simulink model "transfer_function"  (R2023a)
settings: Solver=VariableStepAuto  StartTime=0.0  StopTime=t_simulation  RelTol=1e-3
values from neighbouring files (symbols this model uses):
  A_alpha = -.1    (= -0.1)    [main.m]
  A_beta = 10    [main.m]
  A_wind = -1    [main.m]
  bool_alpha = 0    [main.m]
  bool_beta = 0    [main.m]
  bool_wind = 0    [main.m]
  G_D_sim = table_tf(table_tf.wind_speed==v_wind,:).G_D    [main.m]
  G_D_sim_denominator_1 = table_tf(table_tf.wind_speed==v_wind,:).G_D_denominator{:}(1,1)    [main.m]
  G_D_sim_denominator_2 = table_tf(table_tf.wind_speed==v_wind,:).G_D_denominator{:}(2,1)    [main.m]
  G_D_sim_numerator_1 = table_tf(table_tf.wind_speed==v_wind,:).G_D_numerator{:}(1,1)    [main.m]
  G_D_sim_numerator_2 = table_tf(table_tf.wind_speed==v_wind,:).G_D_numerator{:}(2,1)    [main.m]
  G_S_sim = table_tf(table_tf.wind_speed==v_wind,:).G_S    [main.m]
  G_S_sim_denominator_11 = table_tf(table_tf.wind_speed==v_wind,:).G_S_denominator{:}(1,1)    [main.m]
  G_S_sim_denominator_12 = table_tf(table_tf.wind_speed==v_wind,:).G_S_denominator{:}(1,2)    [main.m]
  G_S_sim_denominator_21 = table_tf(table_tf.wind_speed==v_wind,:).G_S_denominator{:}(2,1)    [main.m]
  G_S_sim_denominator_22 = table_tf(table_tf.wind_speed==v_wind,:).G_S_denominator{:}(2,2)    [main.m]
  G_S_sim_numerator_11 = table_tf(table_tf.wind_speed==v_wind,:).G_S_numerator{:}(1,1)    [main.m]
  G_S_sim_numerator_12 = table_tf(table_tf.wind_speed==v_wind,:).G_S_numerator{:}(1,2)    [main.m]
  G_S_sim_numerator_21 = table_tf(table_tf.wind_speed==v_wind,:).G_S_numerator{:}(2,1)    [main.m]
  G_S_sim_numerator_22 = table_tf(table_tf.wind_speed==v_wind,:).G_S_numerator{:}(2,2)    [main.m]
  PID_11 = PID_Ziegler_Nichols(-G_11,t_linspace)    [main.m]
  pulse_width = 50    [main.m]
  T_delay = 600    [main.m]
  T_period = 1200    [main.m]
libraries: slpidlib x2, cstblocks x2
settings Model: Creator=pascalbock  LastModifiedBy=pascalbock

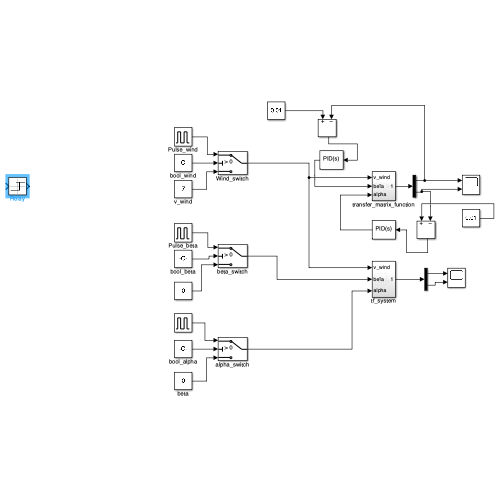
[thumbnail: Simulink's stored preview of the top-level diagram]
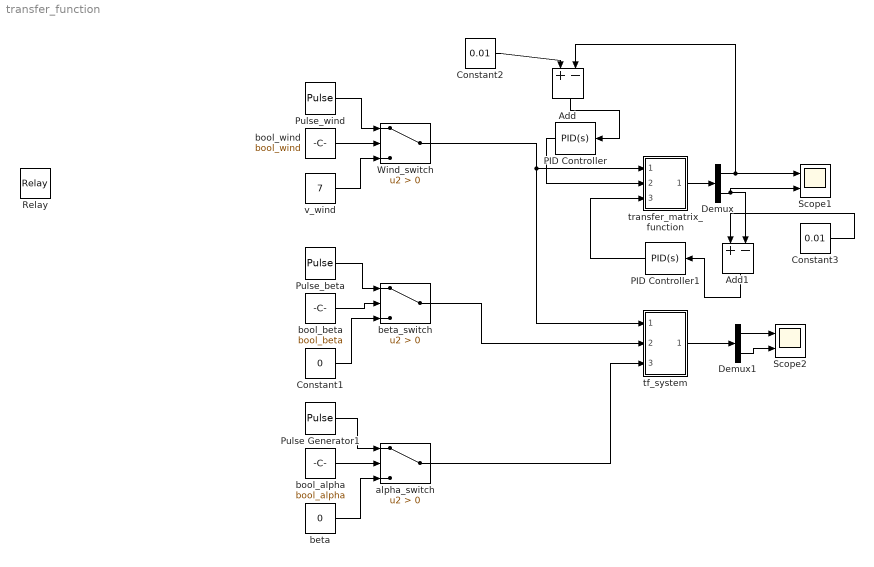
== system transfer_function ==
  Add : Sum  Inputs=+-
  Add1 : Sum  Inputs=+-
  Constant1 : Constant  Value=0
  Constant2 : Constant  Value=0.01
  Constant3 : Constant  Value=0.01
  Demux : Demux  Outputs=2
  Demux1 : Demux  Outputs=2
  PID Controller : slpidlib/PID Controller  Controller=PID  Form=Parallel  TimeDomain=Continuous-time  UseExternalTs=off  SampleTime=-1  IntegratorMethod=Forward Euler  FilterMethod=Forward Euler  ControllerParametersSource=internal  P=PID_11.K_p  I=PID_11.T_I  UseKiTs=off  D=PID_11.T_D  N=100  UseFilter=on  TunerSelectOption=Transfer Function Based (PID Tuner App)  InitialConditionSource=internal  InitialConditionForIntegrator=0  InitialConditionForFilter=0  DifferentiatorICPrevScaledInput=0  ExternalReset=none  TrackingMode=off  Kt=1  LimitOutput=off  SatLimitsSource=internal  UpperSaturationLimit=inf  LowerSaturationLimit=-inf  LinearizeAsGain=on  AntiWindupMode=none  Kb=1  LimitIntegrator=off  UpperIntegratorSaturationLimit=inf  LowerIntegratorSaturationLimit=-inf  POutMin=[]  POutMax=[]  IOutMin=[]  IOutMax=[]  DOutMin=[]  DOutMax=[]  NOutMin=[]  NOutMax=[]  SumOutMin=[]  SumOutMax=[]  SaturationOutMin=[]  SaturationOutMax=[]  PParamMin=[]  PParamMax=[]  IParamMin=[]  IParamMax=[]  DParamMin=[]  DParamMax=[]  NParamMin=[]  NParamMax=[]  KbParamMin=[]  KbParamMax=[]  KtParamMin=[]  KtParamMax=[]  KbOutMin=[]  KbOutMax=[]  KtOutMin=[]  KtOutMax=[]  IntegratorOutMin=[]  IntegratorOutMax=[]  FilterOutMin=[]  FilterOutMax=[]  SumI1OutMin=[]  SumI1OutMax=[]  SumI2OutMin=[]  SumI2OutMax=[]  SumI3OutMin=[]  SumI3OutMax=[]  SumI4OutMin=[]  SumI4OutMax=[]  SumDOutMin=[]  SumDOutMax=[]  DifferentiatorOutMin=[]  DifferentiatorOutMax=[]  FilterDiffOutCoefMin=[]  FilterDiffOutCoefMax=[]  ReciprocalOutMin=[]  ReciprocalOutMax=[]  SumDenOutMin=[]  SumDenOutMax=[]  SumNumOutMin=[]  SumNumOutMax=[]  DivideOutMin=[]  DivideOutMax=[]  UdiffTsProdOutMin=[]  UdiffTsProdOutMax=[]  NTsProdOutMin=[]  NTsProdOutMax=[]  UintegralTsProdOutMin=[]  UintegralTsProdOutMax=[]  UngainTsProdOutMin=[]  UngainTsProdOutMax=[]  ClampingZeroOutDataTypeStr=Inherit: Inherit via back propagation  ClampingZeroOutMin=[]  ClampingZeroOutMax=[]  FilterDenConstantOutDataTypeStr=Inherit: Inherit via back propagation  FilterDenConstantOutMin=[]  FilterDenConstantOutMax=[]  PCopyOutDataTypeStr=Inherit: Inherit via back propagation  PCopyOutMin=[]  PCopyOutMax=[]  NCopyOutDataTypeStr=Inherit: Inherit via back propagation  NCopyOutMin=[]  NCopyOutMax=[]  IntegratorContinuousStateAttributes=''  IntegratorStateMustResolveToSignalObject=off  IntegratorRTWStateStorageClass=Auto  FilterContinuousStateAttributes=''  FilterStateMustResolveToSignalObject=off  FilterRTWStateStorageClass=Auto  ParallelPVariant=InternalParameters  IdealPVariant=Disabled  IVariant=InternalParameters  DVariant=InternalParameters  IntegratorVariant=Continuous  SatVariant=Disabled  AWVariant=Passthrough  PCopyVariant=Disabled  TRVariant=Disabled  FdbkBlocksVariant=Forward  IdealPFdbkVariant=Disabled  SatFdbkVariant=Disabled  DerivativeFilterVariant=ContFilter  NVariant=InternalParameters  NCopyVariant=Disabled  FilterICVariant=InternalICsFilter  IntegratorICVariant=InternalICs  ExternalResetVariant=Disabled  TRSumVariant=Passthrough  SumFdbkVariant=Disabled  SumVariant=Sum_PID  TsampFilterVariant=InternalTs  TsampNgainVariant=Passthrough  TsampIntegralVariant=Disabled_SignalSpec  ExternalSaturationOutDataTypeStr=Inherit: Same as second input
  PID Controller1 : slpidlib/PID Controller  Controller=PID  Form=Parallel  TimeDomain=Continuous-time  UseExternalTs=off  SampleTime=-1  IntegratorMethod=Forward Euler  FilterMethod=Forward Euler  ControllerParametersSource=internal  P=PID_11.K_p  I=PID_11.T_I  UseKiTs=off  D=PID_11.T_D  N=100  UseFilter=on  TunerSelectOption=Transfer Function Based (PID Tuner App)  InitialConditionSource=internal  InitialConditionForIntegrator=0  InitialConditionForFilter=0  DifferentiatorICPrevScaledInput=0  ExternalReset=none  TrackingMode=off  Kt=1  LimitOutput=off  SatLimitsSource=internal  UpperSaturationLimit=inf  LowerSaturationLimit=-inf  LinearizeAsGain=on  AntiWindupMode=none  Kb=1  LimitIntegrator=off  UpperIntegratorSaturationLimit=inf  LowerIntegratorSaturationLimit=-inf  POutMin=[]  POutMax=[]  IOutMin=[]  IOutMax=[]  DOutMin=[]  DOutMax=[]  NOutMin=[]  NOutMax=[]  SumOutMin=[]  SumOutMax=[]  SaturationOutMin=[]  SaturationOutMax=[]  PParamMin=[]  PParamMax=[]  IParamMin=[]  IParamMax=[]  DParamMin=[]  DParamMax=[]  NParamMin=[]  NParamMax=[]  KbParamMin=[]  KbParamMax=[]  KtParamMin=[]  KtParamMax=[]  KbOutMin=[]  KbOutMax=[]  KtOutMin=[]  KtOutMax=[]  IntegratorOutMin=[]  IntegratorOutMax=[]  FilterOutMin=[]  FilterOutMax=[]  SumI1OutMin=[]  SumI1OutMax=[]  SumI2OutMin=[]  SumI2OutMax=[]  SumI3OutMin=[]  SumI3OutMax=[]  SumI4OutMin=[]  SumI4OutMax=[]  SumDOutMin=[]  SumDOutMax=[]  DifferentiatorOutMin=[]  DifferentiatorOutMax=[]  FilterDiffOutCoefMin=[]  FilterDiffOutCoefMax=[]  ReciprocalOutMin=[]  ReciprocalOutMax=[]  SumDenOutMin=[]  SumDenOutMax=[]  SumNumOutMin=[]  SumNumOutMax=[]  DivideOutMin=[]  DivideOutMax=[]  UdiffTsProdOutMin=[]  UdiffTsProdOutMax=[]  NTsProdOutMin=[]  NTsProdOutMax=[]  UintegralTsProdOutMin=[]  UintegralTsProdOutMax=[]  UngainTsProdOutMin=[]  UngainTsProdOutMax=[]  ClampingZeroOutDataTypeStr=Inherit: Inherit via back propagation  ClampingZeroOutMin=[]  ClampingZeroOutMax=[]  FilterDenConstantOutDataTypeStr=Inherit: Inherit via back propagation  FilterDenConstantOutMin=[]  FilterDenConstantOutMax=[]  PCopyOutDataTypeStr=Inherit: Inherit via back propagation  PCopyOutMin=[]  PCopyOutMax=[]  NCopyOutDataTypeStr=Inherit: Inherit via back propagation  NCopyOutMin=[]  NCopyOutMax=[]  IntegratorContinuousStateAttributes=''  IntegratorStateMustResolveToSignalObject=off  IntegratorRTWStateStorageClass=Auto  FilterContinuousStateAttributes=''  FilterStateMustResolveToSignalObject=off  FilterRTWStateStorageClass=Auto  ParallelPVariant=InternalParameters  IdealPVariant=Disabled  IVariant=InternalParameters  DVariant=InternalParameters  IntegratorVariant=Continuous  SatVariant=Disabled  AWVariant=Passthrough  PCopyVariant=Disabled  TRVariant=Disabled  FdbkBlocksVariant=Forward  IdealPFdbkVariant=Disabled  SatFdbkVariant=Disabled  DerivativeFilterVariant=ContFilter  NVariant=InternalParameters  NCopyVariant=Disabled  FilterICVariant=InternalICsFilter  IntegratorICVariant=InternalICs  ExternalResetVariant=Disabled  TRSumVariant=Passthrough  SumFdbkVariant=Disabled  SumVariant=Sum_PID  TsampFilterVariant=InternalTs  TsampNgainVariant=Passthrough  TsampIntegralVariant=Disabled_SignalSpec  ExternalSaturationOutDataTypeStr=Inherit: Same as second input
  Pulse Generator1 : DiscretePulseGenerator  PulseType=Time based  Amplitude=A_alpha  Period=T_period  PulseWidth=pulse_width  PhaseDelay=T_delay
  Pulse_beta : DiscretePulseGenerator  PulseType=Time based  Amplitude=A_beta  Period=T_period  PulseWidth=pulse_width  PhaseDelay=T_delay
  Pulse_wind : DiscretePulseGenerator  PulseType=Time based  Amplitude=A_wind  Period=T_period  PulseWidth=pulse_width  PhaseDelay=T_delay
  Relay : Relay
  Scope1 : Scope  NumInputPorts=2
  Scope2 : Scope  NumInputPorts=2
  Wind_switch : Switch  Criteria=u2 > Threshold  SaturateOnIntegerOverflow=off  InputSameDT=off
  alpha_switch : Switch  Criteria=u2 > Threshold  SaturateOnIntegerOverflow=off  InputSameDT=off
  beta : Constant  Value=0
  beta_switch : Switch  Criteria=u2 > Threshold  SaturateOnIntegerOverflow=off  InputSameDT=off
  bool_alpha : Constant  Value=bool_alpha
  bool_beta : Constant  Value=bool_beta
  bool_wind : Constant  Value=bool_wind
  tf_system : Subsystem
  transfer_matrix_function : Subsystem
  v_wind : Constant  Value=7
  wires:
  transfer_matrix_function/1(Out1) -> Demux/1
  Demux/1 -> Add/2, Scope1/1
  Demux/2 -> Add1/2, Scope1/2
  Pulse_wind/1 -> Wind_switch/1
  v_wind/1 -> Wind_switch/3
  bool_wind/1 -> Wind_switch/2
  bool_alpha/1 -> alpha_switch/2
  beta/1 -> alpha_switch/3
  Pulse_beta/1 -> beta_switch/1
  Pulse Generator1/1 -> alpha_switch/1
  bool_beta/1 -> beta_switch/2
  Wind_switch/1 -> transfer_matrix_function/1(v_wind), tf_system/1(v_wind)
  beta_switch/1 -> tf_system/2(beta)
  alpha_switch/1 -> tf_system/3(alpha)
  Constant1/1 -> beta_switch/3
  tf_system/1(Out1) -> Demux1/1
  Demux1/1 -> Scope2/1
  Demux1/2 -> Scope2/2
  Constant2/1 -> Add/1
  Add/1 -> PID Controller/1
  PID Controller/1 -> transfer_matrix_function/2(beta)
  Add1/1 -> PID Controller1/1
  PID Controller1/1 -> transfer_matrix_function/3(alpha)
  Constant3/1 -> Add1/1

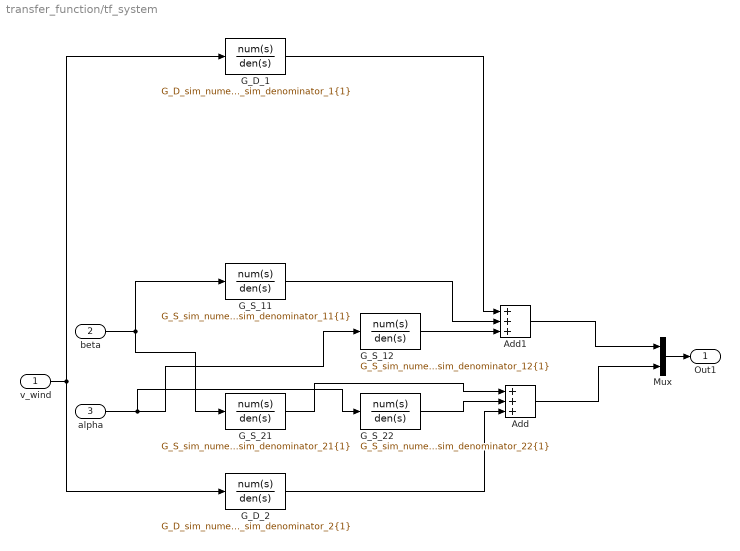
== system transfer_function/tf_system ==
  v_wind : Inport
  beta : Inport  Port=2
  alpha : Inport  Port=3
  Add : Sum  Inputs=+++
  Add1 : Sum  Inputs=+++
  G_D_1 : TransferFcn  Numerator=G_D_sim_numerator_1{1}  Denominator=G_D_sim_denominator_1{1}
  G_D_2 : TransferFcn  Numerator=G_D_sim_numerator_2{1}  Denominator=G_D_sim_denominator_2{1}
  G_S_11 : TransferFcn  Numerator=G_S_sim_numerator_11{1}  Denominator=G_S_sim_denominator_11{1}
  G_S_12 : TransferFcn  Numerator=G_S_sim_numerator_12{1}  Denominator=G_S_sim_denominator_12{1}
  G_S_21 : TransferFcn  Numerator=G_S_sim_numerator_21{1}  Denominator=G_S_sim_denominator_21{1}
  G_S_22 : TransferFcn  Numerator=G_S_sim_numerator_22{1}  Denominator=G_S_sim_denominator_22{1}
  Mux : Mux  Inputs=2
  Out1 : Outport
  wires:
  alpha/1 -> G_S_22/1, G_S_12/1
  G_S_11/1 -> Add1/2
  G_S_12/1 -> Add1/3
  G_S_21/1 -> Add/1
  G_S_22/1 -> Add/2
  v_wind/1 -> G_D_2/1, G_D_1/1
  G_D_1/1 -> Add1/1
  G_D_2/1 -> Add/3
  Add1/1 -> Mux/1
  Add/1 -> Mux/2
  Mux/1 -> Out1/1
  beta/1 -> G_S_11/1, G_S_21/1

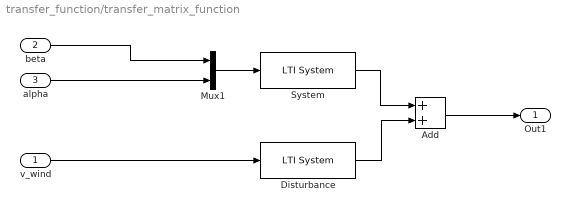
== system transfer_function/transfer_matrix_function ==
  v_wind : Inport
  beta : Inport  Port=2
  alpha : Inport  Port=3
  Add : Sum
  Disturbance : cstblocks/LTI System  sys=G_D_sim{1}  IC=[]
  Mux1 : Mux  Inputs=2
  System : cstblocks/LTI System  sys=G_S_sim{1}  IC=[]
  Out1 : Outport
  wires:
  Add/1 -> Out1/1
  Disturbance/1 -> Add/2
  System/1 -> Add/1
  Mux1/1 -> System/1
  alpha/1 -> Mux1/2
  v_wind/1 -> Disturbance/1
  beta/1 -> Mux1/1
